simulink model "p4_system_arch_master"  (R2020a)
settings: Solver=VariableStepAuto  StartTime=0.0  StopTime=10.0  RelTol=1e-3
(part 6 of 11)

== system p4_system_arch_master/System 10 : Electrical Distribution System /10.2 LV Distribution System /10.2.1	Internal LV Loom System/10.2.1.1	Inverter to Motor LV loom system ==
  10.2.1.1.01	Motor LV loom to inverter PCB connector : Subsystem
      settings: PortSchema="{\"entries\":[{\"content\":{\"headerSize\":26,\"margin\":15,\"minimumSpacing\":25,\"sides\":[{\"content\":{\"connectorIds\":[]},\"type\":\"ConnectorPlacement.EquallySpacedRectSide\",\"uuid\":\"f8ee33a9-954f-44c6-a821-b5353f3278fa\"},{\"content\":{\"connectorIds\":[],\"side\":\"RIGHT\"},\"type\":\"ConnectorPlacement.EquallySpacedRectSide\",\"uuid\":\"385f1e4f-1c89-4afc-9c19-76a078cf90bc\"},{\"content\":{\"connectorIds\":[],\"side\":\"TOP\"},\"type\":\"ConnectorPlacement.EquallySpacedRectSide\",\"uuid\":\"fc91fa49-46f5-4ba7-960e-7bda5e0416d1\"}]},\"type\":\"ConnectorPlacement.EquallySpacedConnector\",\"uuid\":\"4bf08bc6-c7ce-47fb-af04-cd9d2b5f8092\"}],\"packageUris\":[\"http://schema.mathworks.com/mf0/Connector/19700101\"],\"version\":\"1.0\"}"
  PT100 #1 Wire System : Subsystem
      settings: PortSchema="{\"entries\":[{\"content\":{\"headerSize\":26,\"margin\":15,\"minimumSpacing\":25,\"sides\":[{\"content\":{\"connectorIds\":[]},\"type\":\"ConnectorPlacement.EquallySpacedRectSide\",\"uuid\":\"f8ee33a9-954f-44c6-a821-b5353f3278fa\"},{\"content\":{\"connectorIds\":[],\"side\":\"RIGHT\"},\"type\":\"ConnectorPlacement.EquallySpacedRectSide\",\"uuid\":\"385f1e4f-1c89-4afc-9c19-76a078cf90bc\"},{\"content\":{\"connectorIds\":[],\"side\":\"TOP\"},\"type\":\"ConnectorPlacement.EquallySpacedRectSide\",\"uuid\":\"fc91fa49-46f5-4ba7-960e-7bda5e0416d1\"}]},\"type\":\"ConnectorPlacement.EquallySpacedConnector\",\"uuid\":\"4bf08bc6-c7ce-47fb-af04-cd9d2b5f8092\"}],\"packageUris\":[\"http://schema.mathworks.com/mf0/Connector/19700101\"],\"version\":\"1.0\"}"
  PT100 #2 Wire System : Subsystem
      settings: PortSchema="{\"entries\":[{\"content\":{\"headerSize\":26,\"margin\":15,\"minimumSpacing\":25,\"sides\":[{\"content\":{\"connectorIds\":[]},\"type\":\"ConnectorPlacement.EquallySpacedRectSide\",\"uuid\":\"f8ee33a9-954f-44c6-a821-b5353f3278fa\"},{\"content\":{\"connectorIds\":[],\"side\":\"RIGHT\"},\"type\":\"ConnectorPlacement.EquallySpacedRectSide\",\"uuid\":\"385f1e4f-1c89-4afc-9c19-76a078cf90bc\"},{\"content\":{\"connectorIds\":[],\"side\":\"TOP\"},\"type\":\"ConnectorPlacement.EquallySpacedRectSide\",\"uuid\":\"fc91fa49-46f5-4ba7-960e-7bda5e0416d1\"}]},\"type\":\"ConnectorPlacement.EquallySpacedConnector\",\"uuid\":\"4bf08bc6-c7ce-47fb-af04-cd9d2b5f8092\"}],\"packageUris\":[\"http://schema.mathworks.com/mf0/Connector/19700101\"],\"version\":\"1.0\"}"
  Resolver sensor System : Subsystem
      settings: PortSchema="{\"entries\":[{\"content\":{\"headerSize\":26,\"margin\":15,\"minimumSpacing\":25,\"sides\":[{\"content\":{\"connectorIds\":[]},\"type\":\"ConnectorPlacement.EquallySpacedRectSide\",\"uuid\":\"f8ee33a9-954f-44c6-a821-b5353f3278fa\"},{\"content\":{\"connectorIds\":[],\"side\":\"RIGHT\"},\"type\":\"ConnectorPlacement.EquallySpacedRectSide\",\"uuid\":\"385f1e4f-1c89-4afc-9c19-76a078cf90bc\"},{\"content\":{\"connectorIds\":[],\"side\":\"TOP\"},\"type\":\"ConnectorPlacement.EquallySpacedRectSide\",\"uuid\":\"fc91fa49-46f5-4ba7-960e-7bda5e0416d1\"}]},\"type\":\"ConnectorPlacement.EquallySpacedConnector\",\"uuid\":\"4bf08bc6-c7ce-47fb-af04-cd9d2b5f8092\"}],\"packageUris\":[\"http://schema.mathworks.com/mf0/Connector/19700101\"],\"version\":\"1.0\"}"

== system p4_system_arch_master/System 10 : Electrical Distribution System /10.2 LV Distribution System /10.2.1	Internal LV Loom System/10.2.1.2	Inverter to Inverter LV connector loom system ==
  10.2.1.2.01	Inverter LV external connector : Subsystem
      settings: PortSchema="{\"entries\":[{\"content\":{\"headerSize\":26,\"margin\":15,\"minimumSpacing\":25,\"sides\":[{\"content\":{\"connectorIds\":[]},\"type\":\"ConnectorPlacement.EquallySpacedRectSide\",\"uuid\":\"f8ee33a9-954f-44c6-a821-b5353f3278fa\"},{\"content\":{\"connectorIds\":[],\"side\":\"RIGHT\"},\"type\":\"ConnectorPlacement.EquallySpacedRectSide\",\"uuid\":\"385f1e4f-1c89-4afc-9c19-76a078cf90bc\"},{\"content\":{\"connectorIds\":[],\"side\":\"TOP\"},\"type\":\"ConnectorPlacement.EquallySpacedRectSide\",\"uuid\":\"fc91fa49-46f5-4ba7-960e-7bda5e0416d1\"}]},\"type\":\"ConnectorPlacement.EquallySpacedConnector\",\"uuid\":\"4bf08bc6-c7ce-47fb-af04-cd9d2b5f8092\"}],\"packageUris\":[\"http://schema.mathworks.com/mf0/Connector/19700101\"],\"version\":\"1.0\"}"
  10.2.1.2.02	Inverter internal loom to PCB connector : Subsystem
      settings: PortSchema="{\"entries\":[{\"content\":{\"headerSize\":26,\"margin\":15,\"minimumSpacing\":25,\"sides\":[{\"content\":{\"connectorIds\":[]},\"type\":\"ConnectorPlacement.EquallySpacedRectSide\",\"uuid\":\"f8ee33a9-954f-44c6-a821-b5353f3278fa\"},{\"content\":{\"connectorIds\":[],\"side\":\"RIGHT\"},\"type\":\"ConnectorPlacement.EquallySpacedRectSide\",\"uuid\":\"385f1e4f-1c89-4afc-9c19-76a078cf90bc\"},{\"content\":{\"connectorIds\":[],\"side\":\"TOP\"},\"type\":\"ConnectorPlacement.EquallySpacedRectSide\",\"uuid\":\"fc91fa49-46f5-4ba7-960e-7bda5e0416d1\"}]},\"type\":\"ConnectorPlacement.EquallySpacedConnector\",\"uuid\":\"4bf08bc6-c7ce-47fb-af04-cd9d2b5f8092\"}],\"packageUris\":[\"http://schema.mathworks.com/mf0/Connector/19700101\"],\"version\":\"1.0\"}"
  Inverter Internal Wires : Subsystem
      settings: PortSchema="{\"entries\":[{\"content\":{\"headerSize\":26,\"margin\":15,\"minimumSpacing\":25,\"sides\":[{\"content\":{\"connectorIds\":[]},\"type\":\"ConnectorPlacement.EquallySpacedRectSide\",\"uuid\":\"f8ee33a9-954f-44c6-a821-b5353f3278fa\"},{\"content\":{\"connectorIds\":[],\"side\":\"RIGHT\"},\"type\":\"ConnectorPlacement.EquallySpacedRectSide\",\"uuid\":\"385f1e4f-1c89-4afc-9c19-76a078cf90bc\"},{\"content\":{\"connectorIds\":[],\"side\":\"TOP\"},\"type\":\"ConnectorPlacement.EquallySpacedRectSide\",\"uuid\":\"fc91fa49-46f5-4ba7-960e-7bda5e0416d1\"}]},\"type\":\"ConnectorPlacement.EquallySpacedConnector\",\"uuid\":\"4bf08bc6-c7ce-47fb-af04-cd9d2b5f8092\"}],\"packageUris\":[\"http://schema.mathworks.com/mf0/Connector/19700101\"],\"version\":\"1.0\"}"

== system p4_system_arch_master/System 10 : Electrical Distribution System /10.2 LV Distribution System /10.2.1	Internal LV Loom System/10.2.1.3	Internal LV loom restraining system ==
  10.2.1.3.1	Cable clips : Subsystem
      settings: PortSchema="{\"entries\":[{\"content\":{\"headerSize\":26,\"margin\":15,\"minimumSpacing\":25,\"sides\":[{\"content\":{\"connectorIds\":[]},\"type\":\"ConnectorPlacement.EquallySpacedRectSide\",\"uuid\":\"f8ee33a9-954f-44c6-a821-b5353f3278fa\"},{\"content\":{\"connectorIds\":[],\"side\":\"RIGHT\"},\"type\":\"ConnectorPlacement.EquallySpacedRectSide\",\"uuid\":\"385f1e4f-1c89-4afc-9c19-76a078cf90bc\"},{\"content\":{\"connectorIds\":[],\"side\":\"TOP\"},\"type\":\"ConnectorPlacement.EquallySpacedRectSide\",\"uuid\":\"fc91fa49-46f5-4ba7-960e-7bda5e0416d1\"}]},\"type\":\"ConnectorPlacement.EquallySpacedConnector\",\"uuid\":\"4bf08bc6-c7ce-47fb-af04-cd9d2b5f8092\"}],\"packageUris\":[\"http://schema.mathworks.com/mf0/Connector/19700101\"],\"version\":\"1.0\"}"

== system p4_system_arch_master/System 10 : Electrical Distribution System /10.2 LV Distribution System /10.2.2	External LV Loom System/10.2.2.1	External LV loom connectors system ==
  "10.2.2.1.01\tMain LV connector IDU to vehicle " : Subsystem
      settings: PortSchema="{\"entries\":[{\"content\":{\"headerSize\":26,\"margin\":15,\"minimumSpacing\":25,\"sides\":[{\"content\":{\"connectorIds\":[]},\"type\":\"ConnectorPlacement.EquallySpacedRectSide\",\"uuid\":\"f8ee33a9-954f-44c6-a821-b5353f3278fa\"},{\"content\":{\"connectorIds\":[],\"side\":\"RIGHT\"},\"type\":\"ConnectorPlacement.EquallySpacedRectSide\",\"uuid\":\"385f1e4f-1c89-4afc-9c19-76a078cf90bc\"},{\"content\":{\"connectorIds\":[],\"side\":\"TOP\"},\"type\":\"ConnectorPlacement.EquallySpacedRectSide\",\"uuid\":\"fc91fa49-46f5-4ba7-960e-7bda5e0416d1\"}]},\"type\":\"ConnectorPlacement.EquallySpacedConnector\",\"uuid\":\"4bf08bc6-c7ce-47fb-af04-cd9d2b5f8092\"}],\"packageUris\":[\"http://schema.mathworks.com/mf0/Connector/19700101\"],\"version\":\"1.0\"}"
  10.2.2.1.02	Inverter cable connector : Subsystem
      settings: PortSchema="{\"entries\":[{\"content\":{\"headerSize\":26,\"margin\":15,\"minimumSpacing\":25,\"sides\":[{\"content\":{\"connectorIds\":[]},\"type\":\"ConnectorPlacement.EquallySpacedRectSide\",\"uuid\":\"f8ee33a9-954f-44c6-a821-b5353f3278fa\"},{\"content\":{\"connectorIds\":[],\"side\":\"RIGHT\"},\"type\":\"ConnectorPlacement.EquallySpacedRectSide\",\"uuid\":\"385f1e4f-1c89-4afc-9c19-76a078cf90bc\"},{\"content\":{\"connectorIds\":[],\"side\":\"TOP\"},\"type\":\"ConnectorPlacement.EquallySpacedRectSide\",\"uuid\":\"fc91fa49-46f5-4ba7-960e-7bda5e0416d1\"}]},\"type\":\"ConnectorPlacement.EquallySpacedConnector\",\"uuid\":\"4bf08bc6-c7ce-47fb-af04-cd9d2b5f8092\"}],\"packageUris\":[\"http://schema.mathworks.com/mf0/Connector/19700101\"],\"version\":\"1.0\"}"
  10.2.2.1.03	I/O module X1 cable connector : Subsystem
      settings: PortSchema="{\"entries\":[{\"content\":{\"headerSize\":26,\"margin\":15,\"minimumSpacing\":25,\"sides\":[{\"content\":{\"connectorIds\":[]},\"type\":\"ConnectorPlacement.EquallySpacedRectSide\",\"uuid\":\"f8ee33a9-954f-44c6-a821-b5353f3278fa\"},{\"content\":{\"connectorIds\":[],\"side\":\"RIGHT\"},\"type\":\"ConnectorPlacement.EquallySpacedRectSide\",\"uuid\":\"385f1e4f-1c89-4afc-9c19-76a078cf90bc\"},{\"content\":{\"connectorIds\":[],\"side\":\"TOP\"},\"type\":\"ConnectorPlacement.EquallySpacedRectSide\",\"uuid\":\"fc91fa49-46f5-4ba7-960e-7bda5e0416d1\"}]},\"type\":\"ConnectorPlacement.EquallySpacedConnector\",\"uuid\":\"4bf08bc6-c7ce-47fb-af04-cd9d2b5f8092\"}],\"packageUris\":[\"http://schema.mathworks.com/mf0/Connector/19700101\"],\"version\":\"1.0\"}"
  10.2.2.1.04	I/O module X2 cable connector : Subsystem
      settings: PortSchema="{\"entries\":[{\"content\":{\"headerSize\":26,\"margin\":15,\"minimumSpacing\":25,\"sides\":[{\"content\":{\"connectorIds\":[]},\"type\":\"ConnectorPlacement.EquallySpacedRectSide\",\"uuid\":\"f8ee33a9-954f-44c6-a821-b5353f3278fa\"},{\"content\":{\"connectorIds\":[],\"side\":\"RIGHT\"},\"type\":\"ConnectorPlacement.EquallySpacedRectSide\",\"uuid\":\"385f1e4f-1c89-4afc-9c19-76a078cf90bc\"},{\"content\":{\"connectorIds\":[],\"side\":\"TOP\"},\"type\":\"ConnectorPlacement.EquallySpacedRectSide\",\"uuid\":\"fc91fa49-46f5-4ba7-960e-7bda5e0416d1\"}]},\"type\":\"ConnectorPlacement.EquallySpacedConnector\",\"uuid\":\"4bf08bc6-c7ce-47fb-af04-cd9d2b5f8092\"}],\"packageUris\":[\"http://schema.mathworks.com/mf0/Connector/19700101\"],\"version\":\"1.0\"}"
  10.2.2.1.05	Oil temperature sensor connector : Subsystem
      settings: PortSchema="{\"entries\":[{\"content\":{\"headerSize\":26,\"margin\":15,\"minimumSpacing\":25,\"sides\":[{\"content\":{\"connectorIds\":[]},\"type\":\"ConnectorPlacement.EquallySpacedRectSide\",\"uuid\":\"f8ee33a9-954f-44c6-a821-b5353f3278fa\"},{\"content\":{\"connectorIds\":[],\"side\":\"RIGHT\"},\"type\":\"ConnectorPlacement.EquallySpacedRectSide\",\"uuid\":\"385f1e4f-1c89-4afc-9c19-76a078cf90bc\"},{\"content\":{\"connectorIds\":[],\"side\":\"TOP\"},\"type\":\"ConnectorPlacement.EquallySpacedRectSide\",\"uuid\":\"fc91fa49-46f5-4ba7-960e-7bda5e0416d1\"}]},\"type\":\"ConnectorPlacement.EquallySpacedConnector\",\"uuid\":\"4bf08bc6-c7ce-47fb-af04-cd9d2b5f8092\"}],\"packageUris\":[\"http://schema.mathworks.com/mf0/Connector/19700101\"],\"version\":\"1.0\"}"
  10.2.2.1.06	Input speed sensor connector : Subsystem
      settings: PortSchema="{\"entries\":[{\"content\":{\"headerSize\":26,\"margin\":15,\"minimumSpacing\":25,\"sides\":[{\"content\":{\"connectorIds\":[]},\"type\":\"ConnectorPlacement.EquallySpacedRectSide\",\"uuid\":\"f8ee33a9-954f-44c6-a821-b5353f3278fa\"},{\"content\":{\"connectorIds\":[],\"side\":\"RIGHT\"},\"type\":\"ConnectorPlacement.EquallySpacedRectSide\",\"uuid\":\"385f1e4f-1c89-4afc-9c19-76a078cf90bc\"},{\"content\":{\"connectorIds\":[],\"side\":\"TOP\"},\"type\":\"ConnectorPlacement.EquallySpacedRectSide\",\"uuid\":\"fc91fa49-46f5-4ba7-960e-7bda5e0416d1\"}]},\"type\":\"ConnectorPlacement.EquallySpacedConnector\",\"uuid\":\"4bf08bc6-c7ce-47fb-af04-cd9d2b5f8092\"}],\"packageUris\":[\"http://schema.mathworks.com/mf0/Connector/19700101\"],\"version\":\"1.0\"}"
  10.2.2.1.07	Output speed sensor connector : Subsystem
      settings: PortSchema="{\"entries\":[{\"content\":{\"headerSize\":26,\"margin\":15,\"minimumSpacing\":25,\"sides\":[{\"content\":{\"connectorIds\":[]},\"type\":\"ConnectorPlacement.EquallySpacedRectSide\",\"uuid\":\"f8ee33a9-954f-44c6-a821-b5353f3278fa\"},{\"content\":{\"connectorIds\":[],\"side\":\"RIGHT\"},\"type\":\"ConnectorPlacement.EquallySpacedRectSide\",\"uuid\":\"385f1e4f-1c89-4afc-9c19-76a078cf90bc\"},{\"content\":{\"connectorIds\":[],\"side\":\"TOP\"},\"type\":\"ConnectorPlacement.EquallySpacedRectSide\",\"uuid\":\"fc91fa49-46f5-4ba7-960e-7bda5e0416d1\"}]},\"type\":\"ConnectorPlacement.EquallySpacedConnector\",\"uuid\":\"4bf08bc6-c7ce-47fb-af04-cd9d2b5f8092\"}],\"packageUris\":[\"http://schema.mathworks.com/mf0/Connector/19700101\"],\"version\":\"1.0\"}"
  "10.2.2.1.08\tShifting actuator Cable terminal \"+\"" : Subsystem
      settings: PortSchema="{\"entries\":[{\"content\":{\"headerSize\":26,\"margin\":15,\"minimumSpacing\":25,\"sides\":[{\"content\":{\"connectorIds\":[]},\"type\":\"ConnectorPlacement.EquallySpacedRectSide\",\"uuid\":\"f8ee33a9-954f-44c6-a821-b5353f3278fa\"},{\"content\":{\"connectorIds\":[],\"side\":\"RIGHT\"},\"type\":\"ConnectorPlacement.EquallySpacedRectSide\",\"uuid\":\"385f1e4f-1c89-4afc-9c19-76a078cf90bc\"},{\"content\":{\"connectorIds\":[],\"side\":\"TOP\"},\"type\":\"ConnectorPlacement.EquallySpacedRectSide\",\"uuid\":\"fc91fa49-46f5-4ba7-960e-7bda5e0416d1\"}]},\"type\":\"ConnectorPlacement.EquallySpacedConnector\",\"uuid\":\"4bf08bc6-c7ce-47fb-af04-cd9d2b5f8092\"}],\"packageUris\":[\"http://schema.mathworks.com/mf0/Connector/19700101\"],\"version\":\"1.0\"}"
  "10.2.2.1.09\tShifting actuator Cable terminal \"-\"" : Subsystem
      settings: PortSchema="{\"entries\":[{\"content\":{\"headerSize\":26,\"margin\":15,\"minimumSpacing\":25,\"sides\":[{\"content\":{\"connectorIds\":[]},\"type\":\"ConnectorPlacement.EquallySpacedRectSide\",\"uuid\":\"f8ee33a9-954f-44c6-a821-b5353f3278fa\"},{\"content\":{\"connectorIds\":[],\"side\":\"RIGHT\"},\"type\":\"ConnectorPlacement.EquallySpacedRectSide\",\"uuid\":\"385f1e4f-1c89-4afc-9c19-76a078cf90bc\"},{\"content\":{\"connectorIds\":[],\"side\":\"TOP\"},\"type\":\"ConnectorPlacement.EquallySpacedRectSide\",\"uuid\":\"fc91fa49-46f5-4ba7-960e-7bda5e0416d1\"}]},\"type\":\"ConnectorPlacement.EquallySpacedConnector\",\"uuid\":\"4bf08bc6-c7ce-47fb-af04-cd9d2b5f8092\"}],\"packageUris\":[\"http://schema.mathworks.com/mf0/Connector/19700101\"],\"version\":\"1.0\"}"

== system p4_system_arch_master/System 10 : Electrical Distribution System /10.2 LV Distribution System /10.2.2	External LV Loom System/10.2.2.2	External LV loom wiring system ==
  "Barrel Cam Position Speed Sensor Wires " : Subsystem
      settings: PortSchema="{\"entries\":[{\"content\":{\"headerSize\":26,\"margin\":15,\"minimumSpacing\":25,\"sides\":[{\"content\":{\"connectorIds\":[]},\"type\":\"ConnectorPlacement.EquallySpacedRectSide\",\"uuid\":\"f8ee33a9-954f-44c6-a821-b5353f3278fa\"},{\"content\":{\"connectorIds\":[],\"side\":\"RIGHT\"},\"type\":\"ConnectorPlacement.EquallySpacedRectSide\",\"uuid\":\"385f1e4f-1c89-4afc-9c19-76a078cf90bc\"},{\"content\":{\"connectorIds\":[],\"side\":\"TOP\"},\"type\":\"ConnectorPlacement.EquallySpacedRectSide\",\"uuid\":\"fc91fa49-46f5-4ba7-960e-7bda5e0416d1\"}]},\"type\":\"ConnectorPlacement.EquallySpacedConnector\",\"uuid\":\"4bf08bc6-c7ce-47fb-af04-cd9d2b5f8092\"}],\"packageUris\":[\"http://schema.mathworks.com/mf0/Connector/19700101\"],\"version\":\"1.0\"}"
  "O Module Wires " : Subsystem
      settings: PortSchema="{\"entries\":[{\"content\":{\"headerSize\":26,\"margin\":15,\"minimumSpacing\":25,\"sides\":[{\"content\":{\"connectorIds\":[]},\"type\":\"ConnectorPlacement.EquallySpacedRectSide\",\"uuid\":\"f8ee33a9-954f-44c6-a821-b5353f3278fa\"},{\"content\":{\"connectorIds\":[],\"side\":\"RIGHT\"},\"type\":\"ConnectorPlacement.EquallySpacedRectSide\",\"uuid\":\"385f1e4f-1c89-4afc-9c19-76a078cf90bc\"},{\"content\":{\"connectorIds\":[],\"side\":\"TOP\"},\"type\":\"ConnectorPlacement.EquallySpacedRectSide\",\"uuid\":\"fc91fa49-46f5-4ba7-960e-7bda5e0416d1\"}]},\"type\":\"ConnectorPlacement.EquallySpacedConnector\",\"uuid\":\"4bf08bc6-c7ce-47fb-af04-cd9d2b5f8092\"}],\"packageUris\":[\"http://schema.mathworks.com/mf0/Connector/19700101\"],\"version\":\"1.0\"}"

== system p4_system_arch_master/System 10 : Electrical Distribution System /10.2 LV Distribution System /10.2.2	External LV Loom System/10.2.2.3	External LV loom restraining system ==
  10.2.2.3.1	Cable clips : Subsystem
      settings: PortSchema="{\"entries\":[{\"content\":{\"headerSize\":26,\"margin\":15,\"minimumSpacing\":25,\"sides\":[{\"content\":{\"connectorIds\":[]},\"type\":\"ConnectorPlacement.EquallySpacedRectSide\",\"uuid\":\"f8ee33a9-954f-44c6-a821-b5353f3278fa\"},{\"content\":{\"connectorIds\":[],\"side\":\"RIGHT\"},\"type\":\"ConnectorPlacement.EquallySpacedRectSide\",\"uuid\":\"385f1e4f-1c89-4afc-9c19-76a078cf90bc\"},{\"content\":{\"connectorIds\":[],\"side\":\"TOP\"},\"type\":\"ConnectorPlacement.EquallySpacedRectSide\",\"uuid\":\"fc91fa49-46f5-4ba7-960e-7bda5e0416d1\"}]},\"type\":\"ConnectorPlacement.EquallySpacedConnector\",\"uuid\":\"4bf08bc6-c7ce-47fb-af04-cd9d2b5f8092\"}],\"packageUris\":[\"http://schema.mathworks.com/mf0/Connector/19700101\"],\"version\":\"1.0\"}"

== system p4_system_arch_master/System 10 : Electrical Distribution System /10.3 EMI Protection System /10.3.1 Bearing Protection System /10.3.1.1	Motor Shaft to casing grounding component ==

== system p4_system_arch_master/System 10 : Electrical Distribution System /10.3 EMI Protection System /10.3.4 Earthing Grounding System /10.3.4.0.1	Chassis Earth Braid ==

== system p4_system_arch_master/System 10 : Electrical Distribution System /10.3 EMI Protection System /10.3.4 Earthing Grounding System /10.3.4.0.2	Bolts ==

== system p4_system_arch_master/System 10 : Electrical Distribution System /10.3 EMI Protection System /10.3.4 Earthing Grounding System /10.3.4.0.3	Crimp Fitting #1 ==

== system p4_system_arch_master/System 10 : Electrical Distribution System /10.3 EMI Protection System /10.3.4 Earthing Grounding System /10.3.4.0.4	Crimp Fitting #2 ==

== system p4_system_arch_master/System 2 : Gearbox System/2.1 Torque Multiplication System/2.1.1 Gearset System 1/2.1.1.0.2 Gear ==

== system p4_system_arch_master/System 2 : Gearbox System/2.1 Torque Multiplication System/2.1.2 Gearset System 2/2.1.2.0.2 Gear ==

== system p4_system_arch_master/System 2 : Gearbox System/2.1 Torque Multiplication System/2.1.3 Gearset System 3/2.1.3.0.2 Gear ==

== system p4_system_arch_master/System 2 : Gearbox System/2.1 Torque Multiplication System/2.1.5 Bearings System/Countershaft Bearings ==
  "2.1.6.0.3 B3 (NDE Countershaft Bearing) " : Subsystem
      settings: PortSchema="{\"entries\":[{\"content\":{\"headerSize\":26,\"margin\":15,\"minimumSpacing\":25,\"sides\":[{\"content\":{\"connectorIds\":[]},\"type\":\"ConnectorPlacement.EquallySpacedRectSide\",\"uuid\":\"f8ee33a9-954f-44c6-a821-b5353f3278fa\"},{\"content\":{\"connectorIds\":[],\"side\":\"RIGHT\"},\"type\":\"ConnectorPlacement.EquallySpacedRectSide\",\"uuid\":\"385f1e4f-1c89-4afc-9c19-76a078cf90bc\"},{\"content\":{\"connectorIds\":[],\"side\":\"TOP\"},\"type\":\"ConnectorPlacement.EquallySpacedRectSide\",\"uuid\":\"fc91fa49-46f5-4ba7-960e-7bda5e0416d1\"}]},\"type\":\"ConnectorPlacement.EquallySpacedConnector\",\"uuid\":\"4bf08bc6-c7ce-47fb-af04-cd9d2b5f8092\"}],\"packageUris\":[\"http://schema.mathworks.com/mf0/Connector/19700101\"],\"version\":\"1.0\"}"
  "2.1.6.0.4 B4 (DE Countershaft Bearing) " : Subsystem
      settings: PortSchema="{\"entries\":[{\"content\":{\"headerSize\":26,\"margin\":15,\"minimumSpacing\":25,\"sides\":[{\"content\":{\"connectorIds\":[]},\"type\":\"ConnectorPlacement.EquallySpacedRectSide\",\"uuid\":\"f8ee33a9-954f-44c6-a821-b5353f3278fa\"},{\"content\":{\"connectorIds\":[],\"side\":\"RIGHT\"},\"type\":\"ConnectorPlacement.EquallySpacedRectSide\",\"uuid\":\"385f1e4f-1c89-4afc-9c19-76a078cf90bc\"},{\"content\":{\"connectorIds\":[],\"side\":\"TOP\"},\"type\":\"ConnectorPlacement.EquallySpacedRectSide\",\"uuid\":\"fc91fa49-46f5-4ba7-960e-7bda5e0416d1\"}]},\"type\":\"ConnectorPlacement.EquallySpacedConnector\",\"uuid\":\"4bf08bc6-c7ce-47fb-af04-cd9d2b5f8092\"}],\"packageUris\":[\"http://schema.mathworks.com/mf0/Connector/19700101\"],\"version\":\"1.0\"}"

== system p4_system_arch_master/System 2 : Gearbox System/2.1 Torque Multiplication System/2.1.5 Bearings System/Diff Bearings ==
  "2.1.6.0.1 B1 (NDE DIff Bearing)  " : Subsystem
      settings: PortSchema="{\"entries\":[{\"content\":{\"headerSize\":26,\"margin\":15,\"minimumSpacing\":25,\"sides\":[{\"content\":{\"connectorIds\":[]},\"type\":\"ConnectorPlacement.EquallySpacedRectSide\",\"uuid\":\"f8ee33a9-954f-44c6-a821-b5353f3278fa\"},{\"content\":{\"connectorIds\":[],\"side\":\"RIGHT\"},\"type\":\"ConnectorPlacement.EquallySpacedRectSide\",\"uuid\":\"385f1e4f-1c89-4afc-9c19-76a078cf90bc\"},{\"content\":{\"connectorIds\":[],\"side\":\"TOP\"},\"type\":\"ConnectorPlacement.EquallySpacedRectSide\",\"uuid\":\"fc91fa49-46f5-4ba7-960e-7bda5e0416d1\"}]},\"type\":\"ConnectorPlacement.EquallySpacedConnector\",\"uuid\":\"4bf08bc6-c7ce-47fb-af04-cd9d2b5f8092\"}],\"packageUris\":[\"http://schema.mathworks.com/mf0/Connector/19700101\"],\"version\":\"1.0\"}"
  2.1.6.0.2 B2 (DE DIff Bearing) : Subsystem
      settings: PortSchema="{\"entries\":[{\"content\":{\"headerSize\":26,\"margin\":15,\"minimumSpacing\":25,\"sides\":[{\"content\":{\"connectorIds\":[]},\"type\":\"ConnectorPlacement.EquallySpacedRectSide\",\"uuid\":\"f8ee33a9-954f-44c6-a821-b5353f3278fa\"},{\"content\":{\"connectorIds\":[],\"side\":\"RIGHT\"},\"type\":\"ConnectorPlacement.EquallySpacedRectSide\",\"uuid\":\"385f1e4f-1c89-4afc-9c19-76a078cf90bc\"},{\"content\":{\"connectorIds\":[],\"side\":\"TOP\"},\"type\":\"ConnectorPlacement.EquallySpacedRectSide\",\"uuid\":\"fc91fa49-46f5-4ba7-960e-7bda5e0416d1\"}]},\"type\":\"ConnectorPlacement.EquallySpacedConnector\",\"uuid\":\"4bf08bc6-c7ce-47fb-af04-cd9d2b5f8092\"}],\"packageUris\":[\"http://schema.mathworks.com/mf0/Connector/19700101\"],\"version\":\"1.0\"}"

== system p4_system_arch_master/System 2 : Gearbox System/2.1 Torque Multiplication System/2.1.5 Bearings System/Halfshaft Bearings ==
  "2.1.6.0.10 B7 (NDE Halfshaft Bearing) " : Subsystem
      settings: PortSchema="{\"entries\":[{\"content\":{\"headerSize\":26,\"margin\":15,\"minimumSpacing\":25,\"sides\":[{\"content\":{\"connectorIds\":[]},\"type\":\"ConnectorPlacement.EquallySpacedRectSide\",\"uuid\":\"f8ee33a9-954f-44c6-a821-b5353f3278fa\"},{\"content\":{\"connectorIds\":[],\"side\":\"RIGHT\"},\"type\":\"ConnectorPlacement.EquallySpacedRectSide\",\"uuid\":\"385f1e4f-1c89-4afc-9c19-76a078cf90bc\"},{\"content\":{\"connectorIds\":[],\"side\":\"TOP\"},\"type\":\"ConnectorPlacement.EquallySpacedRectSide\",\"uuid\":\"fc91fa49-46f5-4ba7-960e-7bda5e0416d1\"}]},\"type\":\"ConnectorPlacement.EquallySpacedConnector\",\"uuid\":\"4bf08bc6-c7ce-47fb-af04-cd9d2b5f8092\"}],\"packageUris\":[\"http://schema.mathworks.com/mf0/Connector/19700101\"],\"version\":\"1.0\"}"
  "2.1.6.0.11 B8 (DE Halfshaft Bearing) " : Subsystem
      settings: PortSchema="{\"entries\":[{\"content\":{\"headerSize\":26,\"margin\":15,\"minimumSpacing\":25,\"sides\":[{\"content\":{\"connectorIds\":[]},\"type\":\"ConnectorPlacement.EquallySpacedRectSide\",\"uuid\":\"f8ee33a9-954f-44c6-a821-b5353f3278fa\"},{\"content\":{\"connectorIds\":[],\"side\":\"RIGHT\"},\"type\":\"ConnectorPlacement.EquallySpacedRectSide\",\"uuid\":\"385f1e4f-1c89-4afc-9c19-76a078cf90bc\"},{\"content\":{\"connectorIds\":[],\"side\":\"TOP\"},\"type\":\"ConnectorPlacement.EquallySpacedRectSide\",\"uuid\":\"fc91fa49-46f5-4ba7-960e-7bda5e0416d1\"}]},\"type\":\"ConnectorPlacement.EquallySpacedConnector\",\"uuid\":\"4bf08bc6-c7ce-47fb-af04-cd9d2b5f8092\"}],\"packageUris\":[\"http://schema.mathworks.com/mf0/Connector/19700101\"],\"version\":\"1.0\"}"

== system p4_system_arch_master/System 2 : Gearbox System/2.1 Torque Multiplication System/2.1.5 Bearings System/Input Shaft Bearings ==
  "2.1.6.0.5 B5 (NDE Input Shaft Bearing) " : Subsystem
      settings: PortSchema="{\"entries\":[{\"content\":{\"headerSize\":26,\"margin\":15,\"minimumSpacing\":25,\"sides\":[{\"content\":{\"connectorIds\":[]},\"type\":\"ConnectorPlacement.EquallySpacedRectSide\",\"uuid\":\"f8ee33a9-954f-44c6-a821-b5353f3278fa\"},{\"content\":{\"connectorIds\":[],\"side\":\"RIGHT\"},\"type\":\"ConnectorPlacement.EquallySpacedRectSide\",\"uuid\":\"385f1e4f-1c89-4afc-9c19-76a078cf90bc\"},{\"content\":{\"connectorIds\":[],\"side\":\"TOP\"},\"type\":\"ConnectorPlacement.EquallySpacedRectSide\",\"uuid\":\"fc91fa49-46f5-4ba7-960e-7bda5e0416d1\"}]},\"type\":\"ConnectorPlacement.EquallySpacedConnector\",\"uuid\":\"4bf08bc6-c7ce-47fb-af04-cd9d2b5f8092\"}],\"packageUris\":[\"http://schema.mathworks.com/mf0/Connector/19700101\"],\"version\":\"1.0\"}"
  2.1.6.0.6 B6 (DE Input Shaft Bearing) : Subsystem
      settings: PortSchema="{\"entries\":[{\"content\":{\"headerSize\":26,\"margin\":15,\"minimumSpacing\":25,\"sides\":[{\"content\":{\"connectorIds\":[]},\"type\":\"ConnectorPlacement.EquallySpacedRectSide\",\"uuid\":\"f8ee33a9-954f-44c6-a821-b5353f3278fa\"},{\"content\":{\"connectorIds\":[],\"side\":\"RIGHT\"},\"type\":\"ConnectorPlacement.EquallySpacedRectSide\",\"uuid\":\"385f1e4f-1c89-4afc-9c19-76a078cf90bc\"},{\"content\":{\"connectorIds\":[],\"side\":\"TOP\"},\"type\":\"ConnectorPlacement.EquallySpacedRectSide\",\"uuid\":\"fc91fa49-46f5-4ba7-960e-7bda5e0416d1\"}]},\"type\":\"ConnectorPlacement.EquallySpacedConnector\",\"uuid\":\"4bf08bc6-c7ce-47fb-af04-cd9d2b5f8092\"}],\"packageUris\":[\"http://schema.mathworks.com/mf0/Connector/19700101\"],\"version\":\"1.0\"}"

== system p4_system_arch_master/System 2 : Gearbox System/2.1 Torque Multiplication System/2.1.6 Axial Retention System /2.1.6.0.1 Gs1 Bush  ==

== system p4_system_arch_master/System 2 : Gearbox System/2.1 Torque Multiplication System/2.1.6 Axial Retention System /2.1.6.0.2 Thrust Washer ==

== system p4_system_arch_master/System 2 : Gearbox System/2.1 Torque Multiplication System/2.1.6 Axial Retention System /2.1.6.0.3 Nb2 Washer ==

== system p4_system_arch_master/System 2 : Gearbox System/2.1 Torque Multiplication System/2.1.6 Axial Retention System /2.1.6.0.4 Gs3 Washer ==

== system p4_system_arch_master/System 2 : Gearbox System/2.1 Torque Multiplication System/2.1.6 Axial Retention System /2.1.6.0.7 B6_shim ==

== system p4_system_arch_master/System 2 : Gearbox System/2.1 Torque Multiplication System/2.1.6 Axial Retention System /2.1.6.0.8 Bolts ==

== system p4_system_arch_master/System 2 : Gearbox System/2.1 Torque Multiplication System/2.1.6 Axial Retention System /2.1.7.0.5 B2_shim ==

== system p4_system_arch_master/System 2 : Gearbox System/2.1 Torque Multiplication System/2.1.6 Axial Retention System /2.1.7.0.7 B4_shim ==

== system p4_system_arch_master/System 2 : Gearbox System/2.1 Torque Multiplication System/Shaft System/2.1.4.0.1 Countershaft S1 ==

== system p4_system_arch_master/System 2 : Gearbox System/2.1 Torque Multiplication System/Shaft System/2.1.4.0.2 Input Shaft S2  ==

== system p4_system_arch_master/System 2 : Gearbox System/2.2 Gear Shifting System/Force Transfer System 2.2.2/Fork Fixing System 2.2.2.3  ==
  "Bush 1 Fork 1 2.2.2.3.2 " : Subsystem
      settings: PortSchema="{\"entries\":[{\"content\":{\"headerSize\":26,\"margin\":15,\"minimumSpacing\":25,\"sides\":[{\"content\":{\"connectorIds\":[]},\"type\":\"ConnectorPlacement.EquallySpacedRectSide\",\"uuid\":\"f8ee33a9-954f-44c6-a821-b5353f3278fa\"},{\"content\":{\"connectorIds\":[],\"side\":\"RIGHT\"},\"type\":\"ConnectorPlacement.EquallySpacedRectSide\",\"uuid\":\"385f1e4f-1c89-4afc-9c19-76a078cf90bc\"},{\"content\":{\"connectorIds\":[],\"side\":\"TOP\"},\"type\":\"ConnectorPlacement.EquallySpacedRectSide\",\"uuid\":\"fc91fa49-46f5-4ba7-960e-7bda5e0416d1\"}]},\"type\":\"ConnectorPlacement.EquallySpacedConnector\",\"uuid\":\"4bf08bc6-c7ce-47fb-af04-cd9d2b5f8092\"}],\"packageUris\":[\"http://schema.mathworks.com/mf0/Connector/19700101\"],\"version\":\"1.0\"}"
  "Bush 1 Fork 2 2.2.2.3.4 " : Subsystem
      settings: PortSchema="{\"entries\":[{\"content\":{\"headerSize\":26,\"margin\":15,\"minimumSpacing\":25,\"sides\":[{\"content\":{\"connectorIds\":[]},\"type\":\"ConnectorPlacement.EquallySpacedRectSide\",\"uuid\":\"f8ee33a9-954f-44c6-a821-b5353f3278fa\"},{\"content\":{\"connectorIds\":[],\"side\":\"RIGHT\"},\"type\":\"ConnectorPlacement.EquallySpacedRectSide\",\"uuid\":\"385f1e4f-1c89-4afc-9c19-76a078cf90bc\"},{\"content\":{\"connectorIds\":[],\"side\":\"TOP\"},\"type\":\"ConnectorPlacement.EquallySpacedRectSide\",\"uuid\":\"fc91fa49-46f5-4ba7-960e-7bda5e0416d1\"}]},\"type\":\"ConnectorPlacement.EquallySpacedConnector\",\"uuid\":\"4bf08bc6-c7ce-47fb-af04-cd9d2b5f8092\"}],\"packageUris\":[\"http://schema.mathworks.com/mf0/Connector/19700101\"],\"version\":\"1.0\"}"
  "Bush 2 Fork 1 2.2.2.3.3 " : Subsystem
      settings: PortSchema="{\"entries\":[{\"content\":{\"headerSize\":26,\"margin\":15,\"minimumSpacing\":25,\"sides\":[{\"content\":{\"connectorIds\":[]},\"type\":\"ConnectorPlacement.EquallySpacedRectSide\",\"uuid\":\"f8ee33a9-954f-44c6-a821-b5353f3278fa\"},{\"content\":{\"connectorIds\":[],\"side\":\"RIGHT\"},\"type\":\"ConnectorPlacement.EquallySpacedRectSide\",\"uuid\":\"385f1e4f-1c89-4afc-9c19-76a078cf90bc\"},{\"content\":{\"connectorIds\":[],\"side\":\"TOP\"},\"type\":\"ConnectorPlacement.EquallySpacedRectSide\",\"uuid\":\"fc91fa49-46f5-4ba7-960e-7bda5e0416d1\"}]},\"type\":\"ConnectorPlacement.EquallySpacedConnector\",\"uuid\":\"4bf08bc6-c7ce-47fb-af04-cd9d2b5f8092\"}],\"packageUris\":[\"http://schema.mathworks.com/mf0/Connector/19700101\"],\"version\":\"1.0\"}"
  "Bush 2 Fork 2 2.2.2.3.5 " : Subsystem
      settings: PortSchema="{\"entries\":[{\"content\":{\"headerSize\":26,\"margin\":15,\"minimumSpacing\":25,\"sides\":[{\"content\":{\"connectorIds\":[]},\"type\":\"ConnectorPlacement.EquallySpacedRectSide\",\"uuid\":\"f8ee33a9-954f-44c6-a821-b5353f3278fa\"},{\"content\":{\"connectorIds\":[],\"side\":\"RIGHT\"},\"type\":\"ConnectorPlacement.EquallySpacedRectSide\",\"uuid\":\"385f1e4f-1c89-4afc-9c19-76a078cf90bc\"},{\"content\":{\"connectorIds\":[],\"side\":\"TOP\"},\"type\":\"ConnectorPlacement.EquallySpacedRectSide\",\"uuid\":\"fc91fa49-46f5-4ba7-960e-7bda5e0416d1\"}]},\"type\":\"ConnectorPlacement.EquallySpacedConnector\",\"uuid\":\"4bf08bc6-c7ce-47fb-af04-cd9d2b5f8092\"}],\"packageUris\":[\"http://schema.mathworks.com/mf0/Connector/19700101\"],\"version\":\"1.0\"}"
  "Ground Shaft 2.2.2.3.1 " : Subsystem
      settings: PortSchema="{\"entries\":[{\"content\":{\"headerSize\":26,\"margin\":15,\"minimumSpacing\":25,\"sides\":[{\"content\":{\"connectorIds\":[]},\"type\":\"ConnectorPlacement.EquallySpacedRectSide\",\"uuid\":\"f8ee33a9-954f-44c6-a821-b5353f3278fa\"},{\"content\":{\"connectorIds\":[],\"side\":\"RIGHT\"},\"type\":\"ConnectorPlacement.EquallySpacedRectSide\",\"uuid\":\"385f1e4f-1c89-4afc-9c19-76a078cf90bc\"},{\"content\":{\"connectorIds\":[],\"side\":\"TOP\"},\"type\":\"ConnectorPlacement.EquallySpacedRectSide\",\"uuid\":\"fc91fa49-46f5-4ba7-960e-7bda5e0416d1\"}]},\"type\":\"ConnectorPlacement.EquallySpacedConnector\",\"uuid\":\"4bf08bc6-c7ce-47fb-af04-cd9d2b5f8092\"}],\"packageUris\":[\"http://schema.mathworks.com/mf0/Connector/19700101\"],\"version\":\"1.0\"}"

== system p4_system_arch_master/System 2 : Gearbox System/2.2 Gear Shifting System/Force Transfer System 2.2.2/Gear Shift 1 System 2.2.2.1  ==
  "Fork 1 2.2.2.1.2 " : ModelReference  ModelNameDialog=GearShiftFork  SimulationMode=Normal  ModelReferenceVersion=1.1
      settings: PortSchema="{\"entries\":[{\"content\":{\"headerSize\":38,\"margin\":15,\"minimumSpacing\":25,\"sides\":[{\"content\":{\"connectorIds\":[]},\"type\":\"ConnectorPlacement.EquallySpacedRectSide\",\"uuid\":\"a1de0a4a-4383-4256-97c8-b4b7017d79c3\"},{\"content\":{\"connectorIds\":[],\"side\":\"RIGHT\"},\"type\":\"ConnectorPlacement.EquallySpacedRectSide\",\"uuid\":\"b959f0e1-b665-4773-a9ab-23b80a79bba3\"},{\"content\":{\"connectorIds\":[],\"side\":\"TOP\"},\"type\":\"ConnectorPlacement.EquallySpacedRectSide\",\"uuid\":\"884e98bd-fa8a-4556-86a7-182eb6de8f96\"}]},\"type\":\"ConnectorPlacement.EquallySpacedConnector\",\"uuid\":\"31d5ce3f-6fbe-45a5-a872-1e90bd0aea01\"}],\"packageUris\":[\"http://schema.mathworks.com/mf0/Connector/19700101\"],\"version\":\"1.0\"}"
  "Sleeve 1 2.2.2.1.1 " : Subsystem
      settings: PortSchema="{\"entries\":[{\"content\":{\"headerSize\":26,\"margin\":15,\"minimumSpacing\":25,\"sides\":[{\"content\":{\"connectorIds\":[]},\"type\":\"ConnectorPlacement.EquallySpacedRectSide\",\"uuid\":\"f8ee33a9-954f-44c6-a821-b5353f3278fa\"},{\"content\":{\"connectorIds\":[],\"side\":\"RIGHT\"},\"type\":\"ConnectorPlacement.EquallySpacedRectSide\",\"uuid\":\"385f1e4f-1c89-4afc-9c19-76a078cf90bc\"},{\"content\":{\"connectorIds\":[],\"side\":\"TOP\"},\"type\":\"ConnectorPlacement.EquallySpacedRectSide\",\"uuid\":\"fc91fa49-46f5-4ba7-960e-7bda5e0416d1\"}]},\"type\":\"ConnectorPlacement.EquallySpacedConnector\",\"uuid\":\"4bf08bc6-c7ce-47fb-af04-cd9d2b5f8092\"}],\"packageUris\":[\"http://schema.mathworks.com/mf0/Connector/19700101\"],\"version\":\"1.0\"}"

== system p4_system_arch_master/System 2 : Gearbox System/2.2 Gear Shifting System/Force Transfer System 2.2.2/Gear Shift 2 System 2.2.2.2  ==
  Fork 2 2.2.2.2.2 : ModelReference  ModelNameDialog=GearShiftFork  SimulationMode=Normal  ModelReferenceVersion=1.1
      settings: PortSchema="{\"entries\":[{\"content\":{\"headerSize\":38,\"margin\":15,\"minimumSpacing\":25,\"sides\":[{\"content\":{\"connectorIds\":[]},\"type\":\"ConnectorPlacement.EquallySpacedRectSide\",\"uuid\":\"a1de0a4a-4383-4256-97c8-b4b7017d79c3\"},{\"content\":{\"connectorIds\":[],\"side\":\"RIGHT\"},\"type\":\"ConnectorPlacement.EquallySpacedRectSide\",\"uuid\":\"b959f0e1-b665-4773-a9ab-23b80a79bba3\"},{\"content\":{\"connectorIds\":[],\"side\":\"TOP\"},\"type\":\"ConnectorPlacement.EquallySpacedRectSide\",\"uuid\":\"884e98bd-fa8a-4556-86a7-182eb6de8f96\"}]},\"type\":\"ConnectorPlacement.EquallySpacedConnector\",\"uuid\":\"31d5ce3f-6fbe-45a5-a872-1e90bd0aea01\"}],\"packageUris\":[\"http://schema.mathworks.com/mf0/Connector/19700101\"],\"version\":\"1.0\"}"
  "Sleeve 2 2.2.2.2.1 " : Subsystem
      settings: PortSchema="{\"entries\":[{\"content\":{\"headerSize\":26,\"margin\":15,\"minimumSpacing\":25,\"sides\":[{\"content\":{\"connectorIds\":[]},\"type\":\"ConnectorPlacement.EquallySpacedRectSide\",\"uuid\":\"f8ee33a9-954f-44c6-a821-b5353f3278fa\"},{\"content\":{\"connectorIds\":[],\"side\":\"RIGHT\"},\"type\":\"ConnectorPlacement.EquallySpacedRectSide\",\"uuid\":\"385f1e4f-1c89-4afc-9c19-76a078cf90bc\"},{\"content\":{\"connectorIds\":[],\"side\":\"TOP\"},\"type\":\"ConnectorPlacement.EquallySpacedRectSide\",\"uuid\":\"fc91fa49-46f5-4ba7-960e-7bda5e0416d1\"}]},\"type\":\"ConnectorPlacement.EquallySpacedConnector\",\"uuid\":\"4bf08bc6-c7ce-47fb-af04-cd9d2b5f8092\"}],\"packageUris\":[\"http://schema.mathworks.com/mf0/Connector/19700101\"],\"version\":\"1.0\"}"

== system p4_system_arch_master/System 2 : Gearbox System/2.2 Gear Shifting System/Torque Transfer System 2.2.1 /Actuator Gearbox 2.2.1.1  ==
  "Gear  2.2.1.1.2 " : Subsystem
      settings: PortSchema="{\"entries\":[{\"content\":{\"headerSize\":26,\"margin\":15,\"minimumSpacing\":25,\"sides\":[{\"content\":{\"connectorIds\":[]},\"type\":\"ConnectorPlacement.EquallySpacedRectSide\",\"uuid\":\"f8ee33a9-954f-44c6-a821-b5353f3278fa\"},{\"content\":{\"connectorIds\":[],\"side\":\"RIGHT\"},\"type\":\"ConnectorPlacement.EquallySpacedRectSide\",\"uuid\":\"385f1e4f-1c89-4afc-9c19-76a078cf90bc\"},{\"content\":{\"connectorIds\":[],\"side\":\"TOP\"},\"type\":\"ConnectorPlacement.EquallySpacedRectSide\",\"uuid\":\"fc91fa49-46f5-4ba7-960e-7bda5e0416d1\"}]},\"type\":\"ConnectorPlacement.EquallySpacedConnector\",\"uuid\":\"4bf08bc6-c7ce-47fb-af04-cd9d2b5f8092\"}],\"packageUris\":[\"http://schema.mathworks.com/mf0/Connector/19700101\"],\"version\":\"1.0\"}"
  "Gear Circlip 2.2.1.1.4 " : Subsystem
      settings: PortSchema="{\"entries\":[{\"content\":{\"headerSize\":26,\"margin\":15,\"minimumSpacing\":25,\"sides\":[{\"content\":{\"connectorIds\":[]},\"type\":\"ConnectorPlacement.EquallySpacedRectSide\",\"uuid\":\"f8ee33a9-954f-44c6-a821-b5353f3278fa\"},{\"content\":{\"connectorIds\":[],\"side\":\"RIGHT\"},\"type\":\"ConnectorPlacement.EquallySpacedRectSide\",\"uuid\":\"385f1e4f-1c89-4afc-9c19-76a078cf90bc\"},{\"content\":{\"connectorIds\":[],\"side\":\"TOP\"},\"type\":\"ConnectorPlacement.EquallySpacedRectSide\",\"uuid\":\"fc91fa49-46f5-4ba7-960e-7bda5e0416d1\"}]},\"type\":\"ConnectorPlacement.EquallySpacedConnector\",\"uuid\":\"4bf08bc6-c7ce-47fb-af04-cd9d2b5f8092\"}],\"packageUris\":[\"http://schema.mathworks.com/mf0/Connector/19700101\"],\"version\":\"1.0\"}"
  "Pinion 2.2.1.1.1 " : Subsystem
      settings: PortSchema="{\"entries\":[{\"content\":{\"headerSize\":26,\"margin\":15,\"minimumSpacing\":25,\"sides\":[{\"content\":{\"connectorIds\":[]},\"type\":\"ConnectorPlacement.EquallySpacedRectSide\",\"uuid\":\"f8ee33a9-954f-44c6-a821-b5353f3278fa\"},{\"content\":{\"connectorIds\":[],\"side\":\"RIGHT\"},\"type\":\"ConnectorPlacement.EquallySpacedRectSide\",\"uuid\":\"385f1e4f-1c89-4afc-9c19-76a078cf90bc\"},{\"content\":{\"connectorIds\":[],\"side\":\"TOP\"},\"type\":\"ConnectorPlacement.EquallySpacedRectSide\",\"uuid\":\"fc91fa49-46f5-4ba7-960e-7bda5e0416d1\"}]},\"type\":\"ConnectorPlacement.EquallySpacedConnector\",\"uuid\":\"4bf08bc6-c7ce-47fb-af04-cd9d2b5f8092\"}],\"packageUris\":[\"http://schema.mathworks.com/mf0/Connector/19700101\"],\"version\":\"1.0\"}"
  "Pinion Grub Screw 2.2.1.1.3 " : Subsystem
      settings: PortSchema="{\"entries\":[{\"content\":{\"headerSize\":26,\"margin\":15,\"minimumSpacing\":25,\"sides\":[{\"content\":{\"connectorIds\":[]},\"type\":\"ConnectorPlacement.EquallySpacedRectSide\",\"uuid\":\"f8ee33a9-954f-44c6-a821-b5353f3278fa\"},{\"content\":{\"connectorIds\":[],\"side\":\"RIGHT\"},\"type\":\"ConnectorPlacement.EquallySpacedRectSide\",\"uuid\":\"385f1e4f-1c89-4afc-9c19-76a078cf90bc\"},{\"content\":{\"connectorIds\":[],\"side\":\"TOP\"},\"type\":\"ConnectorPlacement.EquallySpacedRectSide\",\"uuid\":\"fc91fa49-46f5-4ba7-960e-7bda5e0416d1\"}]},\"type\":\"ConnectorPlacement.EquallySpacedConnector\",\"uuid\":\"4bf08bc6-c7ce-47fb-af04-cd9d2b5f8092\"}],\"packageUris\":[\"http://schema.mathworks.com/mf0/Connector/19700101\"],\"version\":\"1.0\"}"

== system p4_system_arch_master/System 2 : Gearbox System/2.2 Gear Shifting System/Torque Transfer System 2.2.1 /Drum Fixing System 2.2.1.3  ==
  "Detent Ball 2.2.1.3.3 " : Subsystem
      settings: PortSchema="{\"entries\":[{\"content\":{\"headerSize\":26,\"margin\":15,\"minimumSpacing\":25,\"sides\":[{\"content\":{\"connectorIds\":[]},\"type\":\"ConnectorPlacement.EquallySpacedRectSide\",\"uuid\":\"f8ee33a9-954f-44c6-a821-b5353f3278fa\"},{\"content\":{\"connectorIds\":[],\"side\":\"RIGHT\"},\"type\":\"ConnectorPlacement.EquallySpacedRectSide\",\"uuid\":\"385f1e4f-1c89-4afc-9c19-76a078cf90bc\"},{\"content\":{\"connectorIds\":[],\"side\":\"TOP\"},\"type\":\"ConnectorPlacement.EquallySpacedRectSide\",\"uuid\":\"fc91fa49-46f5-4ba7-960e-7bda5e0416d1\"}]},\"type\":\"ConnectorPlacement.EquallySpacedConnector\",\"uuid\":\"4bf08bc6-c7ce-47fb-af04-cd9d2b5f8092\"}],\"packageUris\":[\"http://schema.mathworks.com/mf0/Connector/19700101\"],\"version\":\"1.0\"}"
  "Detent Body 2.2.1.3.1 " : Subsystem
      settings: PortSchema="{\"entries\":[{\"content\":{\"headerSize\":26,\"margin\":15,\"minimumSpacing\":25,\"sides\":[{\"content\":{\"connectorIds\":[]},\"type\":\"ConnectorPlacement.EquallySpacedRectSide\",\"uuid\":\"f8ee33a9-954f-44c6-a821-b5353f3278fa\"},{\"content\":{\"connectorIds\":[],\"side\":\"RIGHT\"},\"type\":\"ConnectorPlacement.EquallySpacedRectSide\",\"uuid\":\"385f1e4f-1c89-4afc-9c19-76a078cf90bc\"},{\"content\":{\"connectorIds\":[],\"side\":\"TOP\"},\"type\":\"ConnectorPlacement.EquallySpacedRectSide\",\"uuid\":\"fc91fa49-46f5-4ba7-960e-7bda5e0416d1\"}]},\"type\":\"ConnectorPlacement.EquallySpacedConnector\",\"uuid\":\"4bf08bc6-c7ce-47fb-af04-cd9d2b5f8092\"}],\"packageUris\":[\"http://schema.mathworks.com/mf0/Connector/19700101\"],\"version\":\"1.0\"}"
  "Detent Spring 2.2.1.3.2 " : Subsystem
      settings: PortSchema="{\"entries\":[{\"content\":{\"headerSize\":26,\"margin\":15,\"minimumSpacing\":25,\"sides\":[{\"content\":{\"connectorIds\":[]},\"type\":\"ConnectorPlacement.EquallySpacedRectSide\",\"uuid\":\"f8ee33a9-954f-44c6-a821-b5353f3278fa\"},{\"content\":{\"connectorIds\":[],\"side\":\"RIGHT\"},\"type\":\"ConnectorPlacement.EquallySpacedRectSide\",\"uuid\":\"385f1e4f-1c89-4afc-9c19-76a078cf90bc\"},{\"content\":{\"connectorIds\":[],\"side\":\"TOP\"},\"type\":\"ConnectorPlacement.EquallySpacedRectSide\",\"uuid\":\"fc91fa49-46f5-4ba7-960e-7bda5e0416d1\"}]},\"type\":\"ConnectorPlacement.EquallySpacedConnector\",\"uuid\":\"4bf08bc6-c7ce-47fb-af04-cd9d2b5f8092\"}],\"packageUris\":[\"http://schema.mathworks.com/mf0/Connector/19700101\"],\"version\":\"1.0\"}"

== system p4_system_arch_master/System 2 : Gearbox System/2.2 Gear Shifting System/Torque Transfer System 2.2.1 /Torque to Force Translation 2.2.1.2  ==
  "Drum  2.2.1.2.1 " : Subsystem
      settings: PortSchema="{\"entries\":[{\"content\":{\"headerSize\":26,\"margin\":15,\"minimumSpacing\":25,\"sides\":[{\"content\":{\"connectorIds\":[]},\"type\":\"ConnectorPlacement.EquallySpacedRectSide\",\"uuid\":\"f8ee33a9-954f-44c6-a821-b5353f3278fa\"},{\"content\":{\"connectorIds\":[],\"side\":\"RIGHT\"},\"type\":\"ConnectorPlacement.EquallySpacedRectSide\",\"uuid\":\"385f1e4f-1c89-4afc-9c19-76a078cf90bc\"},{\"content\":{\"connectorIds\":[],\"side\":\"TOP\"},\"type\":\"ConnectorPlacement.EquallySpacedRectSide\",\"uuid\":\"fc91fa49-46f5-4ba7-960e-7bda5e0416d1\"}]},\"type\":\"ConnectorPlacement.EquallySpacedConnector\",\"uuid\":\"4bf08bc6-c7ce-47fb-af04-cd9d2b5f8092\"}],\"packageUris\":[\"http://schema.mathworks.com/mf0/Connector/19700101\"],\"version\":\"1.0\"}"
  "Drum Bearing 1 2.2.1.2.2 " : ModelReference  ModelNameDialog=DrumBearing  SimulationMode=Normal  ModelReferenceVersion=1.1
      settings: PortSchema="{\"entries\":[{\"content\":{\"headerSize\":38,\"margin\":15,\"minimumSpacing\":25,\"sides\":[{\"content\":{\"connectorIds\":[]},\"type\":\"ConnectorPlacement.EquallySpacedRectSide\",\"uuid\":\"a1de0a4a-4383-4256-97c8-b4b7017d79c3\"},{\"content\":{\"connectorIds\":[],\"side\":\"RIGHT\"},\"type\":\"ConnectorPlacement.EquallySpacedRectSide\",\"uuid\":\"b959f0e1-b665-4773-a9ab-23b80a79bba3\"},{\"content\":{\"connectorIds\":[],\"side\":\"TOP\"},\"type\":\"ConnectorPlacement.EquallySpacedRectSide\",\"uuid\":\"884e98bd-fa8a-4556-86a7-182eb6de8f96\"}]},\"type\":\"ConnectorPlacement.EquallySpacedConnector\",\"uuid\":\"31d5ce3f-6fbe-45a5-a872-1e90bd0aea01\"}],\"packageUris\":[\"http://schema.mathworks.com/mf0/Connector/19700101\"],\"version\":\"1.0\"}"
  Drum Bearing 2 2.2.1.2.3 : ModelReference  ModelNameDialog=DrumBearing  SimulationMode=Normal  ModelReferenceVersion=1.1
      settings: PortSchema="{\"entries\":[{\"content\":{\"headerSize\":38,\"margin\":15,\"minimumSpacing\":25,\"sides\":[{\"content\":{\"connectorIds\":[]},\"type\":\"ConnectorPlacement.EquallySpacedRectSide\",\"uuid\":\"a1de0a4a-4383-4256-97c8-b4b7017d79c3\"},{\"content\":{\"connectorIds\":[],\"side\":\"RIGHT\"},\"type\":\"ConnectorPlacement.EquallySpacedRectSide\",\"uuid\":\"b959f0e1-b665-4773-a9ab-23b80a79bba3\"},{\"content\":{\"connectorIds\":[],\"side\":\"TOP\"},\"type\":\"ConnectorPlacement.EquallySpacedRectSide\",\"uuid\":\"884e98bd-fa8a-4556-86a7-182eb6de8f96\"}]},\"type\":\"ConnectorPlacement.EquallySpacedConnector\",\"uuid\":\"31d5ce3f-6fbe-45a5-a872-1e90bd0aea01\"}],\"packageUris\":[\"http://schema.mathworks.com/mf0/Connector/19700101\"],\"version\":\"1.0\"}"
  "Drum Shims 2.2.1.2.4 " : Subsystem
      settings: PortSchema="{\"entries\":[{\"content\":{\"headerSize\":26,\"margin\":15,\"minimumSpacing\":25,\"sides\":[{\"content\":{\"connectorIds\":[]},\"type\":\"ConnectorPlacement.EquallySpacedRectSide\",\"uuid\":\"f8ee33a9-954f-44c6-a821-b5353f3278fa\"},{\"content\":{\"connectorIds\":[],\"side\":\"RIGHT\"},\"type\":\"ConnectorPlacement.EquallySpacedRectSide\",\"uuid\":\"385f1e4f-1c89-4afc-9c19-76a078cf90bc\"},{\"content\":{\"connectorIds\":[],\"side\":\"TOP\"},\"type\":\"ConnectorPlacement.EquallySpacedRectSide\",\"uuid\":\"fc91fa49-46f5-4ba7-960e-7bda5e0416d1\"}]},\"type\":\"ConnectorPlacement.EquallySpacedConnector\",\"uuid\":\"4bf08bc6-c7ce-47fb-af04-cd9d2b5f8092\"}],\"packageUris\":[\"http://schema.mathworks.com/mf0/Connector/19700101\"],\"version\":\"1.0\"}"

== system p4_system_arch_master/System 5 : Enclosure and Sealing System X/5.1 Component Enclosure System/5.1.2 RH Gearbox, Motor and Inverter Enclosure System/5.1.2.0.1 RH Gearbox, Motor and Inverter Casing ==

== system p4_system_arch_master/System 5 : Enclosure and Sealing System X/5.1 Component Enclosure System/5.1.2 RH Gearbox, Motor and Inverter Enclosure System/5.1.2.0.2 NDE Motor Cover ==

== system p4_system_arch_master/System 5 : Enclosure and Sealing System X/5.1 Component Enclosure System/5.1.2 RH Gearbox, Motor and Inverter Enclosure System/5.1.2.0.3 Resolver Cover ==

== system p4_system_arch_master/System 5 : Enclosure and Sealing System X/5.1 Component Enclosure System/5.1.2 RH Gearbox, Motor and Inverter Enclosure System/5.1.2.0.4 Top Inverter Cover ==

== system p4_system_arch_master/System 5 : Enclosure and Sealing System X/5.2 Sealing System/5.2.1 Rotary Seals System/5.2.1.0.1 Differential rotary seal LH (SL1) ==

== system p4_system_arch_master/System 5 : Enclosure and Sealing System X/5.2 Sealing System/5.2.1 Rotary Seals System/5.2.1.0.2 Barrel Cam Rotary Seal (SL4) ==

== system p4_system_arch_master/System 5 : Enclosure and Sealing System X/5.2 Sealing System/5.2.1 Rotary Seals System/5.2.1.0.3 Differential rotary seal RH (SL2) ==

== system p4_system_arch_master/System 5 : Enclosure and Sealing System X/5.2 Sealing System/5.2.1 Rotary Seals System/5.2.1.0.4 Input shaft rotary seal (SL3) ==
